simulink model "TorqueVectoring"  (R2023b)
settings: Solver=VariableStepAuto  StartTime=0.0  StopTime=25  FixedStep=1e-3  RelTol=1e-1  AbsTol=1e-3
libraries: simulink x7, autolibshared x5, fuzblock x5, vehdynlibviscommon x1, sim3dlib x1, sim3dautolib x1
(part 1 of 6)
settings Model: Creator=Admin  LastModifiedBy=Elio
settings SolverCC: AutoScaleAbsTol=off
settings DebuggingCC: UnconnectedInputMsg=warning  UnconnectedOutputMsg=warning  UnconnectedLineMsg=warning  SymbolicDimsDataTypeCodeGenerationDiagnostic=none
settings ModelReferenceCC: EnableRefExpFcnMdlSchedulingChecks=on
settings SFSimCC: CustomCodeUndefinedFunction=UseInterfaceOnly
settings RTWCC: DLArmComputeVersion=19.05
settings SimscapeCC: SimscapeLogType=all  SimscapeLogSimulationStatistics=on  SimscapeLogDataHistory=10000

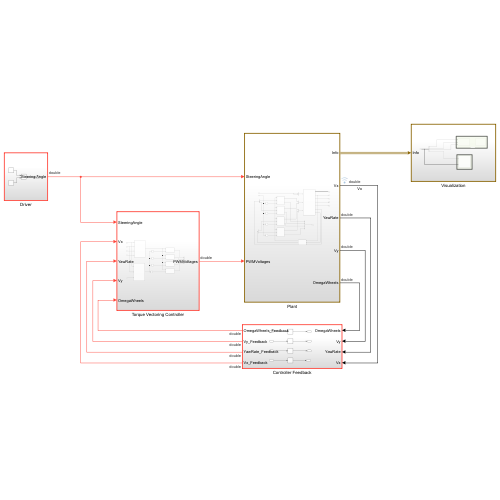
[thumbnail: Simulink's stored preview of the top-level diagram]
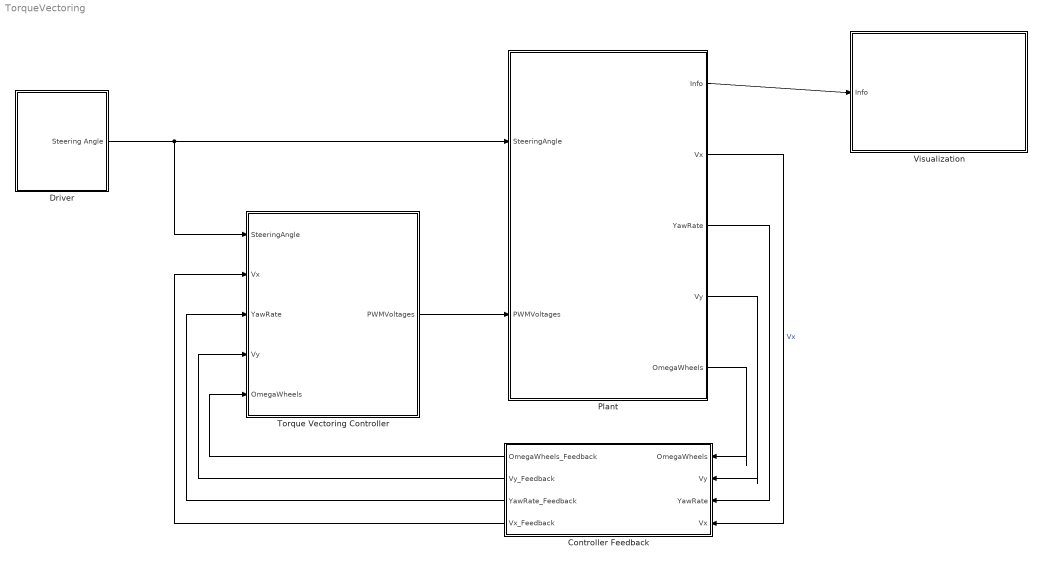
== system TorqueVectoring ==
  Controller Feedback : Subsystem
  Driver : Subsystem
  Plant : Subsystem
  Torque Vectoring Controller : Subsystem
  Visualization : Subsystem
  wires:
  Plant/1(Info) -> Visualization/1(Info)
  Plant/2(Vx) -> Controller Feedback/4(Vx)  "Vx"
  Plant/3(YawRate) -> Controller Feedback/3(YawRate)
  Controller Feedback/4(Vx_Feedback) -> Torque Vectoring Controller/2(Vx)
  Controller Feedback/3(YawRate_Feedback) -> Torque Vectoring Controller/3(YawRate)
  Plant/4(Vy) -> Controller Feedback/2(Vy)
  Controller Feedback/2(Vy_Feedback) -> Torque Vectoring Controller/4(Vy)
  Torque Vectoring Controller/1(PWMVoltages) -> Plant/2(PWMVoltages)
  Driver/1(Steering Angle) -> Torque Vectoring Controller/1(SteeringAngle), Plant/1(SteeringAngle)
  Plant/5(OmegaWheels) -> Controller Feedback/1(OmegaWheels)
  Controller Feedback/1(OmegaWheels_Feedback) -> Torque Vectoring Controller/5(OmegaWheels)

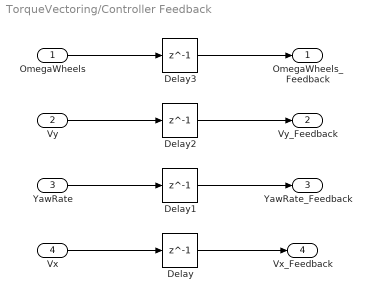
== system TorqueVectoring/Controller Feedback ==
  OmegaWheels : Inport
  Vy : Inport  Port=2
  YawRate : Inport  Port=3
  Vx : Inport  Port=4
  Delay{,1..3} (4 alike) : Delay  DelayLength=1  SampleTime=1e-3
  OmegaWheels_Feedback : Outport
  Vy_Feedback : Outport  Port=2
  YawRate_Feedback : Outport  Port=3
  Vx_Feedback : Outport  Port=4
  wires:
  Vx/1 -> Delay/1
  Delay/1 -> Vx_Feedback/1
  YawRate/1 -> Delay1/1
  Delay1/1 -> YawRate_Feedback/1
  Vy/1 -> Delay2/1
  Delay2/1 -> Vy_Feedback/1
  Delay3/1 -> OmegaWheels_Feedback/1
  OmegaWheels/1 -> Delay3/1

== system TorqueVectoring/Driver ==
  Ramp : simulink/Sources/Ramp  slope=1  start=20  InitialOutput=0
  Ramp1 : simulink/Sources/Ramp  slope=1  start=20.36  InitialOutput=0
  Subtract : Sum  Inputs=+-
  Steering Angle : Outport  SampleTime=1e-3
  wires:
  Ramp/1 -> Subtract/1
  Subtract/1 -> Steering Angle/1
  Ramp1/1 -> Subtract/2

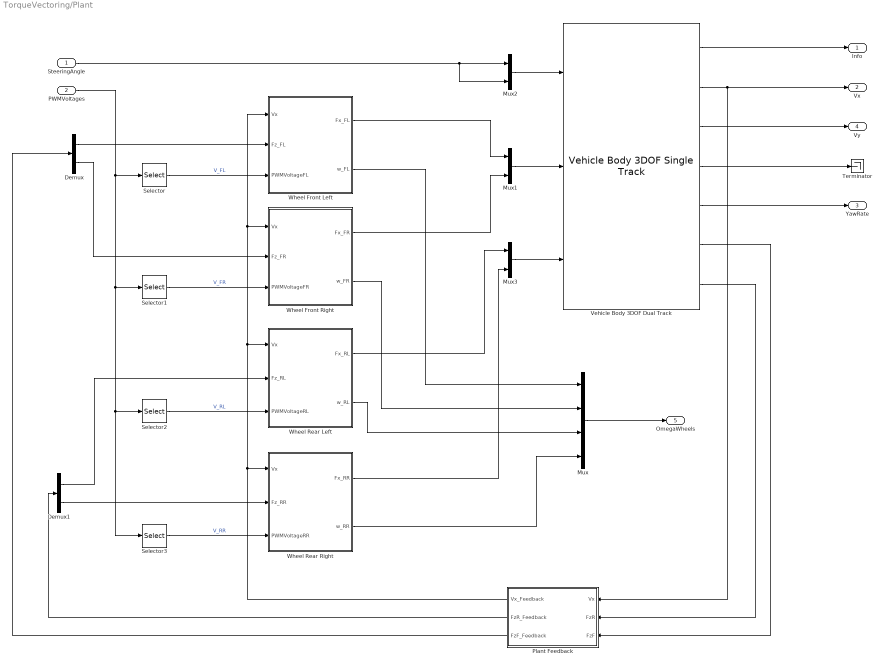
== system TorqueVectoring/Plant ==
  SteeringAngle : Inport
  PWMVoltages : Inport  Port=2
  Demux : Demux  Outputs=2
  Demux1 : Demux  Outputs=2
  Mux : Mux
  Mux1 : Mux  Inputs=2
  Mux2 : Mux  Inputs=2
  Mux3 : Mux  Inputs=2
  Plant Feedback : Subsystem
  Selector : Selector  InputPortWidth=4  IndexOptions=Index vector (dialog)  Indices=1  OutputSizes=1
  Selector1 : Selector  InputPortWidth=4  IndexOptions=Index vector (dialog)  Indices=2  OutputSizes=1
  Selector2 : Selector  InputPortWidth=4  IndexOptions=Index vector (dialog)  Indices=3  OutputSizes=1
  Selector3 : Selector  InputPortWidth=4  IndexOptions=Index vector (dialog)  Indices=4  OutputSizes=1
  Terminator : Terminator
  Vehicle Body 3DOF Dual Track : autolibshared/Vehicle Body 3DOF Single Track  trackMode=Dual  inputMode=External longitudinal forces  frontSteerMode=on  rearSteerMode=off  windMode=off  muMode=off  extFMode=off  extMMode=off  htchFMode=off  htchMMode=off  extXo=off  extpsio=off  extxdoto=off  extro=off  extYo=off  extTamb=off  extydoto=off  aMode=2  NF=2  NR=2  m=1.8  a=0.105  b=0.125  h=0.025  dh=1  hh=0.2  X_o=0  xdot_o=0  CalphaMode=off  sigmaMode=off  d=0  hl=0  w=[0.185,0.185]  Cy_f=70  Cy_r=70  sigma_f=.008  sigma_r=.008  alpha_f_brk=[-.1 .1]  Cy_f_data=[-9e3 9e3]  alpha_r_brk=[-.1 .1]  Cy_r_data=[-9e3 9e3]  Y_o=0  ydot_o=0  Izz=0.0225  psi_o=0  r_o=0  Af=0.03  Cd=0.35  Cl=0.1  Cpm=0.1  beta_w=[0:0.01:0.3]  Cs=[0:0.03:0.9]  Cym=[0:0.01:0.3]  Pabs=101325  Tair=273  g=9.81  mu=1  xdot_tol=.01  Fznom=4.5  Fxtire_sat=7e4  Fytire_sat=7e4  longOff=0  latOff=0  vertOff=0  wrapAng=off
  Wheel Front Left : Subsystem
  Wheel Front Right : Subsystem
  Wheel Rear Left : Subsystem
  Wheel Rear Right : Subsystem
  Info : Outport
  Vx : Outport  Port=2
  YawRate : Outport  Port=3
  Vy : Outport  Port=4
  OmegaWheels : Outport  Port=5
  wires:
  Mux1/1 -> Vehicle Body 3DOF Dual Track/2
  Vehicle Body 3DOF Dual Track/1 -> Info/1
  Vehicle Body 3DOF Dual Track/5 -> YawRate/1
  Vehicle Body 3DOF Dual Track/7 -> Plant Feedback/2(FzR)
  SteeringAngle/1 -> Mux2/2, Mux2/1
  Mux2/1 -> Vehicle Body 3DOF Dual Track/1
  Wheel Front Left/1(Fx_FL) -> Mux1/1
  Wheel Front Right/1(Fx_FR) -> Mux1/2
  Mux3/1 -> Vehicle Body 3DOF Dual Track/3
  Wheel Rear Left/1(Fx_RL) -> Mux3/1
  Wheel Rear Right/1(Fx_RR) -> Mux3/2
  Demux/1 -> Wheel Front Left/2(Fz_FL)
  Demux/2 -> Wheel Front Right/2(Fz_FR)
  Demux1/1 -> Wheel Rear Left/2(Fz_RL)
  Demux1/2 -> Wheel Rear Right/2(Fz_RR)
  Vehicle Body 3DOF Dual Track/2 -> Vx/1, Plant Feedback/1(Vx)
  Vehicle Body 3DOF Dual Track/6 -> Plant Feedback/3(FzF)
  PWMVoltages/1 -> Selector3/1, Selector2/1, Selector1/1, Selector/1
  Selector/1 -> Wheel Front Left/3(PWMVoltageFL)  "V_FL"
  Selector3/1 -> Wheel Rear Right/3(PWMVoltageRR)  "V_RR"
  Selector2/1 -> Wheel Rear Left/3(PWMVoltageRL)  "V_RL"
  Selector1/1 -> Wheel Front Right/3(PWMVoltageFR)  "V_FR"
  Plant Feedback/2(FzR_Feedback) -> Demux1/1
  Plant Feedback/1(Vx_Feedback) -> Wheel Rear Right/1(Vx), Wheel Front Left/1(Vx), Wheel Front Right/1(Vx), Wheel Rear Left/1(Vx)
  Vehicle Body 3DOF Dual Track/3 -> Vy/1
  Plant Feedback/3(FzF_Feedback) -> Demux/1
  Wheel Front Left/2(w_FL) -> Mux/1
  Wheel Front Right/2(w_FR) -> Mux/2
  Wheel Rear Left/2(w_RL) -> Mux/3
  Wheel Rear Right/2(w_RR) -> Mux/4
  Mux/1 -> OmegaWheels/1
  Vehicle Body 3DOF Dual Track/4 -> Terminator/1

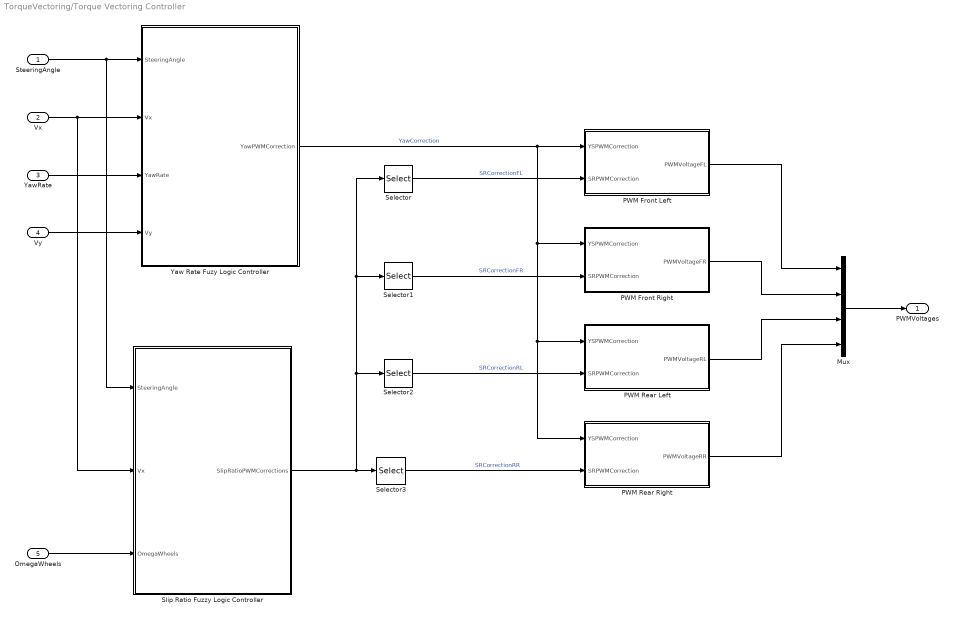
== system TorqueVectoring/Torque Vectoring Controller ==
  SteeringAngle : Inport
  Vx : Inport  Port=2
  YawRate : Inport  Port=3
  Vy : Inport  Port=4
  OmegaWheels : Inport  Port=5
  Mux : Mux
  PWM Front Left : Subsystem
  PWM Front Right : Subsystem
  PWM Rear Left : Subsystem
  PWM Rear Right : Subsystem
  Selector : Selector  InputPortWidth=4  IndexOptions=Index vector (dialog)  Indices=1  OutputSizes=1
  Selector1 : Selector  InputPortWidth=4  IndexOptions=Index vector (dialog)  Indices=2  OutputSizes=1
  Selector2 : Selector  InputPortWidth=4  IndexOptions=Index vector (dialog)  Indices=3  OutputSizes=1
  Selector3 : Selector  InputPortWidth=4  IndexOptions=Index vector (dialog)  Indices=4  OutputSizes=1
  Slip Ratio Fuzzy Logic Controller : Subsystem
  Yaw Rate Fuzy Logic Controller : Subsystem
  PWMVoltages : Outport
  wires:
  YawRate/1 -> Yaw Rate Fuzy Logic Controller/3(YawRate)
  Vy/1 -> Yaw Rate Fuzy Logic Controller/4(Vy)
  Vx/1 -> Slip Ratio Fuzzy Logic Controller/2(Vx), Yaw Rate Fuzy Logic Controller/2(Vx)
  SteeringAngle/1 -> Slip Ratio Fuzzy Logic Controller/1(SteeringAngle), Yaw Rate Fuzy Logic Controller/1(SteeringAngle)
  PWM Front Left/1(PWMVoltageFL) -> Mux/1
  PWM Front Right/1(PWMVoltageFR) -> Mux/2
  PWM Rear Left/1(PWMVoltageRL) -> Mux/3
  PWM Rear Right/1(PWMVoltageRR) -> Mux/4
  Mux/1 -> PWMVoltages/1
  OmegaWheels/1 -> Slip Ratio Fuzzy Logic Controller/3(OmegaWheels)
  Slip Ratio Fuzzy Logic Controller/1(SlipRatioPWMCorrections) -> Selector2/1, Selector/1, Selector1/1, Selector3/1
  Yaw Rate Fuzy Logic Controller/1(YawPWMCorrection) -> PWM Rear Right/1(YSPWMCorrection), PWM Rear Left/1(YSPWMCorrection), PWM Front Right/1(YSPWMCorrection), PWM Front Left/1(YSPWMCorrection)  "YawCorrection"
  Selector1/1 -> PWM Front Right/2(SRPWMCorrection)  "SRCorrectionFR"
  Selector/1 -> PWM Front Left/2(SRPWMCorrection)  "SRCorrectionFL"
  Selector2/1 -> PWM Rear Left/2(SRPWMCorrection)  "SRCorrectionRL"
  Selector3/1 -> PWM Rear Right/2(SRPWMCorrection)  "SRCorrectionRR"

== system TorqueVectoring/Visualization ==
  note: 3D Visualization
  Info : Inport
  2D Visualization : Subsystem
      mask Display: image("visualization.JPG");
  Bus Selector : BusSelector  OutputSignals=InertFrm.Geom.Disp.X,InertFrm.Geom.Disp.Y,InertFrm.Cg.Ang.psi,BdyFrm.FrntAxl.Steer.WhlAngFL
  Simulation 3D Scene Configuration : sim3dlib/Simulation 3D Scene Configuration  Priority=0  Commented=on  ProjectFormat=Default Scenes  SceneDesc=Straight road  ProjectName=C:\Program Files\MATLAB\R2023b\toolbox\shared\sim3d_projects\automotive_project_windows\UE\WindowsNoEditor\VehicleSimulation.exe  ScenePath=/Game/Maps/HwStrght  EnableOpenDRIVE=off  vehTagList={'Custom';'Scene Origin';'SimulinkVehicle1'}  vehTag=SimulinkVehicle1  FreeCameraInitialTranslation=[0, 0, 0]  FreeCameraDefaultInitialTranslation=[-6, 0, 2]  FreeCameraInitialRotation=[0, 0, 0]  FreeCameraDefaultInitialRotation=[0, -15, 0]  OpVisEn=off  Ts=.02  EnableWindow=on  EnableRemoteAccess=off  EnableWeather=off  SunAltitude=40.0  SunAzimuth=90  clouds=10  wind=1  fog=0  rain=0  EnableGeospatial=off  OriginHeight=200  OriginLatitude=40.744652  OriginLongitude=-73.988864  MapStyle=Aerial  AdditionalAssetIDs=[]  UseAdvancedSunSky=off  SolarTime=11  TimeZone=-5  Day=21  Month=9  Year=2022  UseDaylightSavingTime=on  DSTStartDay=10  DSTStartMonth=3  DSTEndDay=3  DSTEndMonth=11  DSTSwitchHour=2  sensorTag=MainCamera1  sensorId=1  sensorName=MainCamera1  mountLoc=Origin  offsetFlag=off  tmountOffset=[0, 0, 0]  rmountOffset=[0, 0, 0]  HorizontalResolution=1280  VerticalResolution=720  HorizontalFOV=60  mountPoint=[0 0 0]  mountOrientation=[0 0 0]  aMode=2  ID=1  GeoTrigger=Inactive
      settings: LibrarySourceBlock=vehdynlibsim3dcore/Simulation 3D Scene Configuration
  Simulation 3D-Vehicle with Ground Following : sim3dautolib/Simulation 3D Vehicle with Ground Following VDBS  Priority=-1  Commented=on  PassVehMesh=Muscle car  MeshPath=/MathWorksSimulation/Vehicles/Muscle/Meshes/SK_MuscleCar.SK_MuscleCar  TrackWidth=0.2  WheelBase=0.35  WheelRadius=0.035  VehColor=Red  InitialPos=[0, 0, 0]  InitialRot=[0, 0, 0]  ActorName=SimulinkVehicle1  VehLightsControl=off  HeadlightColor=[ 1, 1, 1 ]  HighBeamIntensity=100000  LowBeamIntensity=60000  HighBeamConeAngle=1.22  LowBeamConeAngle=1.22  LeftHeadlightOrientation=[ 0, 0 ]  RightHeadlightOrientation=[ 0, 0 ]  BrakelightIntensity=200  ReverselightIntensity=500  SignallightIntensity=500  SignallightPeriod=1  SignalPulseWidth=50  SampleTime=-1  ActorType=SimulinkVehicle  ID=1  aMode=2  ActorTag=SimulinkVehicle1  CoordinateScheme=SAE
      settings: LibrarySourceBlock=vehdynlibsim3d/Simulation 3D Vehicle with Ground Following
  wires:
  Bus Selector/2 -> Simulation 3D-Vehicle with Ground Following/2  "<Y>"
  Bus Selector/1 -> Simulation 3D-Vehicle with Ground Following/1  "<X>"
  Info/1 -> Bus Selector/1, 2D Visualization/2(Info)
  Bus Selector/3 -> Simulation 3D-Vehicle with Ground Following/3  "<psi>"
  Bus Selector/4 -> 2D Visualization/1(SteeringAngle)  "<WhlAngFL>"

== system TorqueVectoring/Plant/Plant Feedback ==
  Vx : Inport
  FzR : Inport  Port=2
  FzF : Inport  Port=3
  Delay : Delay  DelayLength=1
  Delay1 : Delay  DelayLength=1
  Delay2 : Delay  DelayLength=1
  Vx_Feedback : Outport
  FzR_Feedback : Outport  Port=2
  FzF_Feedback : Outport  Port=3
  wires:
  FzR/1 -> Delay/1
  Delay/1 -> FzR_Feedback/1
  FzF/1 -> Delay1/1
  Delay1/1 -> FzF_Feedback/1
  Vx/1 -> Delay2/1
  Delay2/1 -> Vx_Feedback/1
